simulink model "basic_model1"  (R2022b)
settings: Solver=ode45  StartTime=0.0  StopTime=120  RelTol=1e-3
values from neighbouring files (symbols this model uses):
  b = 50    [cruise_control_1.m]    (also in cruise_control_PID.m; engine.m = 0.1)
  m = 1000    [cruise_control_1.m]    (also in cruise_control_PID.m)
settings Model: Creator=sansh  LastModifiedBy=hlubik03
settings SolverCC: AlgebraicLoopSolver=TrustRegion
settings DataIOCC: ReturnWorkspaceOutputs=off
settings DebuggingCC: UnconnectedInputMsg=warning  UnconnectedOutputMsg=warning  UnconnectedLineMsg=warning  SFMachineParentedDataDiag=warning  ArithmeticOperatorsInVariantConditions=warning
settings ModelReferenceCC: EnableRefExpFcnMdlSchedulingChecks=on
settings SFSimCC: SimUseLocalCustomCode=off  CustomCodeUndefinedFunction=UseInterfaceOnly
settings RTWCC: RTWUseLocalCustomCode=off
settings CodeAppCC: StateflowObjectComments=on

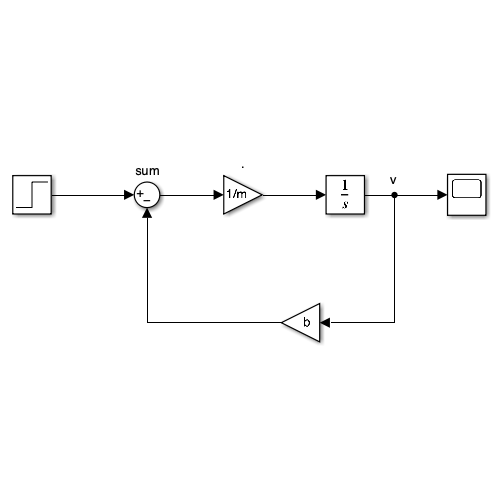
[thumbnail: Simulink's stored preview of the top-level diagram]
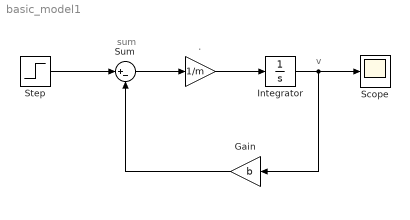
== system basic_model1 ==
  note: v
  note: sum
  . : Gain  Gain=1/m
  Gain : Gain  Gain=b
  Integrator : Integrator
  Scope : Scope
  Step : Step  After=u  SampleTime=0
  Sum : Sum  Inputs=|+-
  wires:
  Integrator/1 -> Gain/1, Scope/1
  ./1 -> Integrator/1
  Sum/1 -> ./1
  Gain/1 -> Sum/2
  Step/1 -> Sum/1
